simulink model "udp_simulation"  (R2020b)
settings: Solver=VariableStepAuto  StartTime=0.0  StopTime=10.0  RelTol=1e-3
undefined symbols (not defined in the file): f
libraries: instrumentlib x4
settings Model: Creator=georg  LastModifiedBy=georg

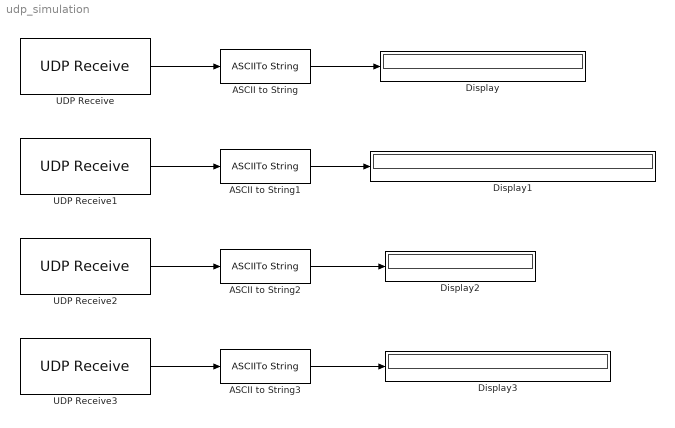
== system udp_simulation ==
  ASCII to String{,1..3} (4 alike) : ASCIIToString
  Display{,1..3} (4 alike) : Display
  UDP Receive : instrumentlib/UDP Receive  Host=localhost  Port=9090  LocalPort=4444  EnablePortSharing=off  GetLatestData=off  DataSize=40  DataType=uint8  ASCIIFormatting=%f,  Terminator=LF  ByteOrder=BigEndian  EnableBlockingMode=on  Timeout=10  SampleTime=0.01  LocalAddress=127.0.0.1
  UDP Receive1 : instrumentlib/UDP Receive  Host=localhost  Port=9090  LocalPort=4443  EnablePortSharing=off  GetLatestData=off  DataSize=49  DataType=uint8  ASCIIFormatting=%f,  Terminator=LF  ByteOrder=BigEndian  EnableBlockingMode=on  Timeout=10  SampleTime=0.01  LocalAddress=127.0.0.1
  UDP Receive2 : instrumentlib/UDP Receive  Host=localhost  Port=9090  LocalPort=4442  EnablePortSharing=off  GetLatestData=off  DataSize=27  DataType=uint8  ASCIIFormatting=%f,  Terminator=LF  ByteOrder=BigEndian  EnableBlockingMode=on  Timeout=10  SampleTime=0.01  LocalAddress=127.0.0.1
  UDP Receive3 : instrumentlib/UDP Receive  Host=localhost  Port=9090  LocalPort=4441  EnablePortSharing=off  GetLatestData=off  DataSize=41  DataType=uint8  ASCIIFormatting=%f,  Terminator=LF  ByteOrder=BigEndian  EnableBlockingMode=on  Timeout=10  SampleTime=0.01  LocalAddress=127.0.0.1
  wires:
  ASCII to String2/1 -> Display2/1
  ASCII to String1/1 -> Display1/1
  ASCII to String/1 -> Display/1
  ASCII to String3/1 -> Display3/1
  UDP Receive/1 -> ASCII to String/1
  UDP Receive1/1 -> ASCII to String1/1
  UDP Receive2/1 -> ASCII to String2/1
  UDP Receive3/1 -> ASCII to String3/1
